simulink model "FM_V6_Zikun"  (R2022b)
settings: Solver=VariableStepAuto  StartTime=0.0  StopTime=1240
values from neighbouring files (symbols this model uses):
  A_fc = 550    [CNV.m]
  A_st = 1.1*A_fc*1E-4*n_cell*0.0012    (= 0.047553)    [CNV.m]
  A_T_rm = 0.005    [CNV.m]
  b11 = 0.005139    [CNV.m]
  b12 = 0.00326    [CNV.m]
  b2 = 350    [CNV.m]
  c1 = 10    [CNV.m]
  c3 = 2    [CNV.m]
  cc = 30    [CNV.m]
  Cd_rm = 0.0124    [CNV.m]
  Cp_air = 1005    [CNV.m]
  Cp_cl = 4180    [CNV.m]
  Cp_st = Cp_Al*1.5    (= 1350)    [CNV.m]
  F = 96485    [CNV.m]
  gamma = 1.4    [CNV.m]
  H_conv_st = 3    [CNV.m]
  i_max = 2.2    [CNV.m]
  k_ca_out = 0.2177*10^(-5)    (= 2.177e-06)    [CNV.m]
  K_sm_out = 0.3629*10^-5    (= 3.629e-06)    [CNV.m]
  kd_cp = 0.01    [CNV.m]
  kd_rm = 0    [CNV.m]
  ki_cp = 0.1    [CNV.m]
  ki_fan = -1E-5    (= -1e-05)    [CNV.m]
  ki_rm = -5E-8    (= -5e-08)    [CNV.m]
  kp_cp = 7.5    [CNV.m]
  kp_fan = -0.5    [CNV.m]
  kp_rm = -8E-7    (= -8e-07)    [CNV.m]
  M_a = 29*10^-3    (= 0.029)    [CNV.m]
  M_H2 = 2*10^-3    (= 0.002)    [CNV.m]
  m_H2_initial = P_atm*V_an/(R_H2*T_atm)    (= 0.00044494386048)    [CNV.m]
  m_H2O_initial = 0.005    [CNV.m]
  M_m_dry = 1.1    [CNV.m]
  M_N2 = 28*10^-3    (= 0.028)    [CNV.m]
  m_N2_initial = P_atm*(1-y_O2)*V_ca/(R_N2*T_atm)    (= 0.00586138039643)    [CNV.m]
  M_O2 = 32*10^-3    (= 0.032)    [CNV.m]
  m_O2_initial = P_atm*y_O2*V_ca/(R_O2*T_atm)    (= 0.00177998712422)    [CNV.m]
  m_st = n_cell*A_fc*t_m*rho_m_dry+(V_ca+V_an)*rho_Al*2.5    (= 87.4506875)    [CNV.m]
  M_v = 18*10^-3    (= 0.018)    [CNV.m]
  n_cell = 655    [CNV.m]
  P_a = P_atm*(1-L*h/T_atm)^(g*M_a/(R*L))    [CNV.m]
  P_atm = 101.25*10^3    (= 101250)    [CNV.m]
  P_ca_ref = 2.5*P_a    [CNV.m]
  phi_a = 0.1    [CNV.m]
  phi_des = 1    [CNV.m]
  R = 8.315    [CNV.m]
  R_a = 286.9    [CNV.m]
  R_H2 = 4124.3    [CNV.m]
  R_N2 = 296.8    [CNV.m]
  R_O2 = 259.8    [CNV.m]
  R_v = 461.5    [CNV.m]
  rho_a = P_a/(R_a*T_a)    [CNV.m]
  rho_H2 = 0.0899    [CNV.m]
  rho_m_dry = 0.002    [CNV.m]
  rho_N2 = 1.165    [CNV.m]
  T_a = T_atm-h*L    [CNV.m]
  T_atm = 298.15    [CNV.m]
  T_cl = 353.15    [CNV.m]
  t_m = 0.01    [CNV.m]
  T_rm = 303.15    [CNV.m]
  T_st_ref = 353.15    [CNV.m]
  V_an = n_cell*A_fc*10^(-4)*0.0005*0.3    (= 0.00540375)    [CNV.m]
  V_ca = n_cell*A_fc*10^(-4)*0.0006*0.3    (= 0.0064845)    [CNV.m]
  V_rm = 0.005    [CNV.m]
  V_sm = 0.02    [CNV.m]
  y_O2_ca_in = 0.21    [CNV.m]
libraries: fl_lib x64, nesl_utility x40, ee_lib x18, fl_ps_legacy_lib x6, SimscapeFluids_lib x5, slpidlib x4, simulink x3, batteryecm_lib x1, autolibshared x1
(part 5 of 6)

== system FM_V6_Zikun/Subsystem/FuelCellStack1/MembraneHydration ==
  I_st : Inport
  T_st : Inport  Port=2
  phi_ca : Inport  Port=3
  phi_an : Inport  Port=4
  3.67-3.70 : MATLAB Function  TreatAsAtomicUnit=on
  3.72-3.73 : MATLAB Function  TreatAsAtomicUnit=on
  3.74 : MATLAB Function  TreatAsAtomicUnit=on
  3.75-3.76 : MATLAB Function  TreatAsAtomicUnit=on
  3.77-3.78 : Gain  Gain=rho_m_dry/M_m_dry
  Add : Sum
  Constant : Constant  Value=n_cell
  Constant1 : Constant  Value=M_v
  Constant2 : Constant  Value=A_fc
  Constant3 : Constant  Value=t_m
  Constant4 : Constant  Value=F
  Demux : Demux  Outputs=2
  Gain : Gain  Gain=1/A_fc
  Mux : Mux  Inputs=2
  Scope : Scope
  lambda_m : Outport
  W_v_mem : Outport  Port=2
  wires:
  Mux/1 -> 3.77-3.78/1
  Demux/1 -> 3.67-3.70/4(c_v_ca)
  Demux/2 -> 3.67-3.70/5(c_v_an)
  3.72-3.73/2(lambda_ca) -> Mux/1
  3.72-3.73/3(lambda_an) -> Mux/2
  3.77-3.78/1 -> Demux/1
  I_st/1 -> Gain/1
  phi_ca/1 -> Add/1, 3.72-3.73/1(phi_ca)
  phi_an/1 -> Add/2, 3.72-3.73/2(phi_an)
  3.67-3.70/1(W_v_mem) -> W_v_mem/1
  3.72-3.73/1(lambda_m) -> 3.74/1(lambda_m), 3.75-3.76/1(lambda_m), lambda_m/1
  3.74/1(n_d) -> 3.67-3.70/1(n_d)
  3.75-3.76/1(D_w) -> 3.67-3.70/3(D_w)
  T_st/1 -> 3.75-3.76/2(T_st)
  Gain/1 -> 3.67-3.70/2(i)
  Constant/1 -> 3.67-3.70/6(n_cell)
  Constant1/1 -> 3.67-3.70/8(M_v)
  Constant2/1 -> 3.67-3.70/7(A_fc)
  Constant3/1 -> 3.67-3.70/9(t_m)
  Constant4/1 -> 3.67-3.70/10(F)
  Add/1 -> Scope/1

== system FM_V6_Zikun/Subsystem/FuelCellStack1/StackVoltage ==
  P_ca : Inport
  P_O2 : Inport  Port=2
  lambda_m : Inport  Port=3
  P_H2 : Inport  Port=4
  P_sat : Inport  Port=5
  T_st : Inport  Port=6
  I_st : Inport  Port=7
  ActivationLoss : Subsystem
  ConcentrationLoss : Subsystem
  Constant : Constant  Value=n_cell
  Demux : Demux
  Gain : Gain  Gain=1/A_fc
  MATLAB Function : MATLAB Function  TreatAsAtomicUnit=on
  Mux : Mux
  NernstVoltage : MATLAB Function  TreatAsAtomicUnit=on
  OhmicLoss : Subsystem
  Pa2Bar : Gain  Gain=0.00001
  Product : Product
  Scope1 : Scope  NumInputPorts=5
  Scope2 : Scope
  Scope3 : Scope  NumInputPorts=4
  To Workspace : ToWorkspace  VariableName=simout  SaveFormat=Timeseries  SampleTime=-1
  VoltageBehaviour : Subsystem  Commented=on
  StackVoltage : Outport
  tag scope: CellVoltage=global, I_den=global
  wires:
  ConcentrationLoss/1(V_conc) -> MATLAB Function/4(V_conc), Scope1/4
  MATLAB Function/1(V_cell) -> Scope1/5, [CellVoltage], Product/1, Scope2/1, To Workspace/1  "V_cell"
  OhmicLoss/1(V_ohm) -> MATLAB Function/3(V_ohm), Scope1/3
  Constant/1 -> Product/2
  Product/1 -> StackVoltage/1
  NernstVoltage/1(E_T_P) -> MATLAB Function/1(E_T_P), Scope1/1
  ActivationLoss/1(V_act) -> MATLAB Function/2(V_act), Scope1/2
  T_st/1 -> ConcentrationLoss/2(T_st), OhmicLoss/2(T_st), ActivationLoss/1(T_st), NernstVoltage/1(T_st)
  lambda_m/1 -> OhmicLoss/3(lambda_m)
  I_st/1 -> Gain/1
  Gain/1 -> [I_den], ConcentrationLoss/1(I_den), ActivationLoss/5(I_den), OhmicLoss/1(I_den)
  P_H2/1 -> Mux/1
  P_O2/1 -> Mux/2
  P_sat/1 -> Mux/4
  Mux/1 -> Pa2Bar/1
  Demux/1 -> NernstVoltage/2(P_H2)
  Demux/2 -> ActivationLoss/4(P_O2), ConcentrationLoss/3(P_O2), NernstVoltage/3(P_O2)
  Demux/3 -> ActivationLoss/2(P_ca)
  Demux/4 -> ConcentrationLoss/4(P_sat), ActivationLoss/3(P_sat)
  Pa2Bar/1 -> Demux/1
  P_ca/1 -> Mux/3

== system FM_V6_Zikun/Subsystem/FuelCellStack1/Thermo ==
  Constant : Constant  Value=n_cell
  MATLAB Function : MATLAB Function  TreatAsAtomicUnit=on
  Scope : Scope  NumInputPorts=2
  wires:
  [I_st] -> MATLAB Function/1(I_st)
  Constant/1 -> MATLAB Function/3(n_cell)
  [CellVoltage] -> MATLAB Function/2(V_cell)
  MATLAB Function/1(P_loss_reac) -> Scope/1
  [P_st] -> Scope/2

== system FM_V6_Zikun/Subsystem/Subsystem2/Subsystem ==
  T_cl_in : Inport
  I_st : Inport  Port=2
  Constant : Constant  Value=0.3
  Constant1 : Constant  Value=Cp_air
  Constant2 : Constant  Value=Cp_cl
  Constant3 : Constant  Value=T_a
  Constant4 : Constant  Value=T_st_ref
  Constant5 : Constant  Value=0
  Constant6 : Constant  Value=10
  Demux : Demux  Outputs=2
  MATLAB Function : MATLAB Function  TreatAsAtomicUnit=on
  MATLAB Function1 : MATLAB Function  TreatAsAtomicUnit=on
  MATLAB Function3 : MATLAB Function  TreatAsAtomicUnit=on
  Minus : Sum  Inputs=+-
  Mux : Mux  Inputs=2
  Mux1 : Mux  Inputs=2
  PID Controller1 : slpidlib/PID Controller  Controller=PID  Form=Parallel  TimeDomain=Continuous-time  UseExternalTs=off  SampleTime=-1  IntegratorMethod=Forward Euler  FilterMethod=Forward Euler  ControllerParametersSource=internal  P=kp_fan  I=ki_fan  UseKiTs=off  D=0  N=100  UseFilter=on  TunerSelectOption=Transfer Function Based (PID Tuner App)  InitialConditionSource=internal  InitialConditionForIntegrator=0  InitialConditionForFilter=0  DifferentiatorICPrevScaledInput=0  ExternalReset=none  TrackingMode=off  Kt=1  LimitOutput=off  SatLimitsSource=internal  UpperSaturationLimit=inf  LowerSaturationLimit=-inf  LinearizeAsGain=on  AntiWindupMode=none  Kb=1  LimitIntegrator=off  UpperIntegratorSaturationLimit=inf  LowerIntegratorSaturationLimit=-inf  POutMin=[]  POutMax=[]  IOutMin=[]  IOutMax=[]  DOutMin=[]  DOutMax=[]  NOutMin=[]  NOutMax=[]  SumOutMin=[]  SumOutMax=[]  SaturationOutMin=[]  SaturationOutMax=[]  PParamMin=[]  PParamMax=[]  IParamMin=[]  IParamMax=[]  DParamMin=[]  DParamMax=[]  NParamMin=[]  NParamMax=[]  KbParamMin=[]  KbParamMax=[]  KtParamMin=[]  KtParamMax=[]  KbOutMin=[]  KbOutMax=[]  KtOutMin=[]  KtOutMax=[]  IntegratorOutMin=[]  IntegratorOutMax=[]  FilterOutMin=[]  FilterOutMax=[]  SumI1OutMin=[]  SumI1OutMax=[]  SumI2OutMin=[]  SumI2OutMax=[]  SumI3OutMin=[]  SumI3OutMax=[]  SumI4OutMin=[]  SumI4OutMax=[]  SumDOutMin=[]  SumDOutMax=[]  DifferentiatorOutMin=[]  DifferentiatorOutMax=[]  FilterDiffOutCoefMin=[]  FilterDiffOutCoefMax=[]  ReciprocalOutMin=[]  ReciprocalOutMax=[]  SumDenOutMin=[]  SumDenOutMax=[]  SumNumOutMin=[]  SumNumOutMax=[]  DivideOutMin=[]  DivideOutMax=[]  UdiffTsProdOutMin=[]  UdiffTsProdOutMax=[]  NTsProdOutMin=[]  NTsProdOutMax=[]  UintegralTsProdOutMin=[]  UintegralTsProdOutMax=[]  UngainTsProdOutMin=[]  UngainTsProdOutMax=[]  ClampingZeroOutDataTypeStr=Inherit: Inherit via back propagation  ClampingZeroOutMin=[]  ClampingZeroOutMax=[]  FilterDenConstantOutDataTypeStr=Inherit: Inherit via back propagation  FilterDenConstantOutMin=[]  FilterDenConstantOutMax=[]  PCopyOutDataTypeStr=Inherit: Inherit via back propagation  PCopyOutMin=[]  PCopyOutMax=[]  NCopyOutDataTypeStr=Inherit: Inherit via back propagation  NCopyOutMin=[]  NCopyOutMax=[]  IntegratorContinuousStateAttributes=''  IntegratorStateMustResolveToSignalObject=off  IntegratorRTWStateStorageClass=Auto  FilterContinuousStateAttributes=''  FilterStateMustResolveToSignalObject=off  FilterRTWStateStorageClass=Auto  ParallelPVariant=InternalParameters  IdealPVariant=Disabled  IVariant=InternalParameters  DVariant=InternalParameters  IntegratorVariant=Continuous  SatVariant=Disabled  AWVariant=Passthrough  PCopyVariant=Disabled  TRVariant=Disabled  FdbkBlocksVariant=Forward  IdealPFdbkVariant=Disabled  SatFdbkVariant=Disabled  DerivativeFilterVariant=ContFilter  NVariant=InternalParameters  NCopyVariant=Disabled  FilterICVariant=InternalICsFilter  IntegratorICVariant=InternalICs  ExternalResetVariant=Disabled  TRSumVariant=Passthrough  SumFdbkVariant=Disabled  SumVariant=Sum_PID  TsampFilterVariant=InternalTs  TsampNgainVariant=Passthrough  TsampIntegralVariant=Passthrough  ExternalSaturationOutDataTypeStr=Inherit: Same as second input
  PID Controller2 : slpidlib/PID Controller  Controller=PID  Form=Parallel  TimeDomain=Continuous-time  UseExternalTs=off  SampleTime=-1  IntegratorMethod=Forward Euler  FilterMethod=Forward Euler  ControllerParametersSource=internal  P=-0.5  I=-1E-3  UseKiTs=off  D=0  N=100  UseFilter=on  TunerSelectOption=Transfer Function Based (PID Tuner App)  InitialConditionSource=internal  InitialConditionForIntegrator=0  InitialConditionForFilter=0  DifferentiatorICPrevScaledInput=0  ExternalReset=none  TrackingMode=off  Kt=1  LimitOutput=off  SatLimitsSource=internal  UpperSaturationLimit=inf  LowerSaturationLimit=-inf  LinearizeAsGain=on  AntiWindupMode=none  Kb=1  LimitIntegrator=off  UpperIntegratorSaturationLimit=inf  LowerIntegratorSaturationLimit=-inf  POutMin=[]  POutMax=[]  IOutMin=[]  IOutMax=[]  DOutMin=[]  DOutMax=[]  NOutMin=[]  NOutMax=[]  SumOutMin=[]  SumOutMax=[]  SaturationOutMin=[]  SaturationOutMax=[]  PParamMin=[]  PParamMax=[]  IParamMin=[]  IParamMax=[]  DParamMin=[]  DParamMax=[]  NParamMin=[]  NParamMax=[]  KbParamMin=[]  KbParamMax=[]  KtParamMin=[]  KtParamMax=[]  KbOutMin=[]  KbOutMax=[]  KtOutMin=[]  KtOutMax=[]  IntegratorOutMin=[]  IntegratorOutMax=[]  FilterOutMin=[]  FilterOutMax=[]  SumI1OutMin=[]  SumI1OutMax=[]  SumI2OutMin=[]  SumI2OutMax=[]  SumI3OutMin=[]  SumI3OutMax=[]  SumI4OutMin=[]  SumI4OutMax=[]  SumDOutMin=[]  SumDOutMax=[]  DifferentiatorOutMin=[]  DifferentiatorOutMax=[]  FilterDiffOutCoefMin=[]  FilterDiffOutCoefMax=[]  ReciprocalOutMin=[]  ReciprocalOutMax=[]  SumDenOutMin=[]  SumDenOutMax=[]  SumNumOutMin=[]  SumNumOutMax=[]  DivideOutMin=[]  DivideOutMax=[]  UdiffTsProdOutMin=[]  UdiffTsProdOutMax=[]  NTsProdOutMin=[]  NTsProdOutMax=[]  UintegralTsProdOutMin=[]  UintegralTsProdOutMax=[]  UngainTsProdOutMin=[]  UngainTsProdOutMax=[]  ClampingZeroOutDataTypeStr=Inherit: Inherit via back propagation  ClampingZeroOutMin=[]  ClampingZeroOutMax=[]  FilterDenConstantOutDataTypeStr=Inherit: Inherit via back propagation  FilterDenConstantOutMin=[]  FilterDenConstantOutMax=[]  PCopyOutDataTypeStr=Inherit: Inherit via back propagation  PCopyOutMin=[]  PCopyOutMax=[]  NCopyOutDataTypeStr=Inherit: Inherit via back propagation  NCopyOutMin=[]  NCopyOutMax=[]  IntegratorContinuousStateAttributes=''  IntegratorStateMustResolveToSignalObject=off  IntegratorRTWStateStorageClass=Auto  FilterContinuousStateAttributes=''  FilterStateMustResolveToSignalObject=off  FilterRTWStateStorageClass=Auto  ParallelPVariant=InternalParameters  IdealPVariant=Disabled  IVariant=InternalParameters  DVariant=InternalParameters  IntegratorVariant=Continuous  SatVariant=Disabled  AWVariant=Passthrough  PCopyVariant=Disabled  TRVariant=Disabled  FdbkBlocksVariant=Forward  IdealPFdbkVariant=Disabled  SatFdbkVariant=Disabled  DerivativeFilterVariant=ContFilter  NVariant=InternalParameters  NCopyVariant=Disabled  FilterICVariant=InternalICsFilter  IntegratorICVariant=InternalICs  ExternalResetVariant=Disabled  TRSumVariant=Passthrough  SumFdbkVariant=Disabled  SumVariant=Sum_PID  TsampFilterVariant=InternalTs  TsampNgainVariant=Passthrough  TsampIntegralVariant=Passthrough  ExternalSaturationOutDataTypeStr=Inherit: Same as second input
  Plus : Sum  Inputs=+-
  Saturation : Saturate  UpperLimit=5  LowerLimit=0
  Scope : Scope  NumInputPorts=2
  Switch : Switch  Criteria=u2 > Threshold  Threshold=20  SaturateOnIntegerOverflow=off  InputSameDT=off
  To Workspace1 : ToWorkspace  VariableName=W_cl_rad  SaveFormat=Timeseries  SampleTime=-1
  To Workspace7 : ToWorkspace  VariableName=W_air_rad  SaveFormat=Timeseries  SampleTime=-1
  P_pump_loss : Outport
  P_fan_loss : Outport  Port=2
  P_cl : Outport  Port=3
  wires:
  T_cl_in/1 -> MATLAB Function/3(T_cl_in), Plus/2, MATLAB Function3/2(T_st)
  Constant4/1 -> Minus/1, MATLAB Function3/1(T_st_ref)
  MATLAB Function1/2(P_pump_loss) -> P_pump_loss/1
  MATLAB Function1/1(P_fan_loss) -> P_fan_loss/1
  MATLAB Function/1(P_cl) -> P_cl/1
  Constant/1 -> MATLAB Function/4(nu_rad)
  Constant1/1 -> MATLAB Function/5(Cp_a)
  Constant2/1 -> MATLAB Function/6(Cp_cl)
  Constant3/1 -> MATLAB Function/7(T_a_in)
  MATLAB Function3/2(e_fan) -> PID Controller1/1
  PID Controller1/1 -> Mux/2
  MATLAB Function3/1(W_cl) -> Mux/1
  I_st/1 -> Switch/2
  Mux/1 -> Switch/1
  Demux/1 -> Saturation/1
  Demux/2 -> To Workspace7/1, MATLAB Function1/1(W_a), Scope/2, MATLAB Function/2(W_a)
  Switch/1 -> Demux/1
  Mux1/1 -> Switch/3
  Constant5/1 -> Mux1/2
  PID Controller2/1 -> Mux1/1
  Plus/1 -> PID Controller2/1
  Saturation/1 -> To Workspace1/1, MATLAB Function1/2(W_cl), Scope/1, MATLAB Function/1(W_cl)
  Minus/1 -> Plus/1
  Constant6/1 -> Minus/2

== system FM_V6_Zikun/Subsystem/Subsystem2/ThermoCalc ==
  I_st : Inport
  P_st : Inport  Port=2
  P_cl : Inport  Port=3
  Add : Sum  Inputs=+---
  Constant : Constant  Value=F
  Constant1 : Constant  Value=n_cell
  Constant2 : Constant  Value=T_a
  Constant6 : Constant  Value=H_conv_st
  Constant7 : Constant  Value=A_st
  Gain : Gain  Gain=1/(m_st*Cp_st)
  Integrator : Integrator  InitialCondition=T_a
  P_conv : MATLAB Function  TreatAsAtomicUnit=on
  P_tot : MATLAB Function  TreatAsAtomicUnit=on
  Saturation1 : Saturate  Commented=through  UpperLimit=400  LowerLimit=T_a
  Scope : Scope  NumInputPorts=4
  T_st : Outport
  P_tot_st : Outport  Port=2
  wires:
  P_cl/1 -> Scope/3, Add/3
  Constant6/1 -> P_conv/1(k_conv)
  Constant2/1 -> P_conv/3(T_a)
  P_st/1 -> Scope/2, Add/2
  Constant7/1 -> P_conv/2(A_st)
  Gain/1 -> Integrator/1
  Constant1/1 -> P_tot/3(n_cell)
  Integrator/1 -> P_conv/4(T_st), Saturation1/1
  P_conv/1(P_conv) -> Scope/4, Add/4
  Add/1 -> Gain/1
  P_tot/1(P_tot) -> Scope/1, Add/1, P_tot_st/1
  Constant/1 -> P_tot/2(F)
  I_st/1 -> P_tot/1(I_st)
  Saturation1/1 -> T_st/1

== system FM_V6_Zikun/Subsystem/Supply Manifold/Manifold Filling ==
  W_cp : Inport
  T_cp_out : Inport  Port=2
  W_sm_out : Inport  Port=3
  Constant : Constant  Value=T_atm
  Constant1 : Constant  Value=gamma
  Constant2 : Constant  Value=R_a
  Constant3 : Constant  Value=V_sm
  Integrator : Integrator  InitialCondition=P_atm
  Integrator1 : Integrator
  MATLAB Function : MATLAB Function  TreatAsAtomicUnit=on
  MATLAB Function1 : MATLAB Function  TreatAsAtomicUnit=on
  MATLAB Function2 : MATLAB Function  TreatAsAtomicUnit=on
  Switch : Switch  Criteria=u2 > Threshold  SaturateOnIntegerOverflow=off  InputSameDT=off
  p_sm : Outport
  T_sm : Outport  Port=2
  wires:
  W_cp/1 -> MATLAB Function1/1(W_cp), MATLAB Function/1(W_cp)
  T_cp_out/1 -> MATLAB Function1/2(T_cp_out)
  MATLAB Function1/1(d_p_sm_dt) -> Integrator/1
  MATLAB Function2/1(T_sm) -> Switch/1, Switch/2, T_sm/1
  Integrator/1 -> p_sm/1, MATLAB Function2/2(p_sm)
  MATLAB Function/1(d_m_sm_dt) -> Integrator1/1
  W_sm_out/1 -> MATLAB Function/2(W_sm_out), MATLAB Function1/3(W_sm_out)
  Integrator1/1 -> MATLAB Function2/1(m_sm)
  Constant/1 -> Switch/3
  Switch/1 -> MATLAB Function1/4(T_sm)
  Constant1/1 -> MATLAB Function1/5(gamma)
  Constant2/1 -> MATLAB Function1/6(R_a), MATLAB Function2/4(R_a)
  Constant3/1 -> MATLAB Function1/7(V_sm), MATLAB Function2/3(V_sm)

== system FM_V6_Zikun/Subsystem/Supply Manifold/Nozzle ==
  P_ca : Inport
  P_sm : Inport  Port=2
  Constant : Constant  Value=K_sm_out
  MATLAB Function : MATLAB Function  TreatAsAtomicUnit=on
  W_sm_out : Outport
  wires:
  P_sm/1 -> MATLAB Function/1(P_sm)
  P_ca/1 -> MATLAB Function/2(P_ca)
  MATLAB Function/1(W_sm_out) -> W_sm_out/1
  Constant/1 -> MATLAB Function/3(k_sm_out)

== system FM_V6_Zikun/D/Subsystem/Electric Pump System/Temperature measurement1 ==
  Tamb : Inport
  Convective Heat Transfer : fl_lib/Thermal/Thermal Elements/Convective Heat Transfer  thermal_type=foundation.enum.constant_variable.constant  area=0.1 m^2  heat_tr_coeff=5 W/(m^2 * K)  min_heat_tr_coeff=1e-3 W/(K*m^2)  T_specify=off  T_priority=None  T=0 K  T_nominal_specify=off  T_nominal_unit=K  T_nominal_value=1  Q_specify=off  Q_priority=None  Q=0 J/s  Q_nominal_specify=off  Q_nominal_unit=J/s  Q_nominal_value=1
  PS-Simulink Converter1 : nesl_utility/PS-Simulink Converter  PhysicalDomain=network_engine_domain  SubClassName=ps_output  LeftPortType=input  RightPortType=output  PseudoPeriodic=off  Frequencies=[]  VectorFormat=1-D array  Unit=degC  AffineConversion=on
  Simulink-PS Converter1 : nesl_utility/Simulink-PS Converter  PhysicalDomain=network_engine_domain  SubClassName=ps_input  LeftPortType=input  RightPortType=output  PseudoPeriodic=off  Frequencies=[]  NoiseDistribution=none  NoiseParameters=[]  Unit=degC  AffineConversion=on  FilteringAndDerivatives=zero  SimscapeFilterOrder=1  InputFilterTimeConstant=0.001  UdotUserProvided=1
  Temperature Sensor : fl_lib/Thermal/Thermal Sensors/Temperature Sensor
  Temperature Source : fl_lib/Thermal/Thermal Sources/Controlled Temperature Source
  Thermal Reference : fl_lib/Thermal/Thermal Elements/Thermal Reference
  H : PMIOPort  Side=Right
  T : Outport  VectorParamsAs1DForOutWhenUnconnected=off
  wires:
  Tamb/1 -> Simulink-PS Converter1/1
  PS-Simulink Converter1/1 -> T/1  "Temperature [degC]"
  connections:
  Convective Heat Transfer/RConn1 -- Temperature Source/LConn1
  Temperature Sensor/RConn2 -- PS-Simulink Converter1/LConn1
  Temperature Sensor/LConn1 -- H/RConn1 -- Convective Heat Transfer/LConn1
  Simulink-PS Converter1/RConn1 -- Temperature Source/RConn1
  Thermal Reference/LConn1 -- Temperature Sensor/RConn1 -- Temperature Source/RConn2

== system FM_V6_Zikun/D/Subsystem/Electric Pump System/Temperature measurement2 ==
  Tamb : Inport
  Convective Heat Transfer : fl_lib/Thermal/Thermal Elements/Convective Heat Transfer  thermal_type=foundation.enum.constant_variable.constant  area=0.1 m^2  heat_tr_coeff=5 W/(m^2 * K)  min_heat_tr_coeff=1e-3 W/(K*m^2)  T_specify=off  T_priority=None  T=0 K  T_nominal_specify=off  T_nominal_unit=K  T_nominal_value=1  Q_specify=off  Q_priority=None  Q=0 J/s  Q_nominal_specify=off  Q_nominal_unit=J/s  Q_nominal_value=1
  PS-Simulink Converter1 : nesl_utility/PS-Simulink Converter  PhysicalDomain=network_engine_domain  SubClassName=ps_output  LeftPortType=input  RightPortType=output  PseudoPeriodic=off  Frequencies=[]  VectorFormat=1-D array  Unit=degC  AffineConversion=on
  Simulink-PS Converter1 : nesl_utility/Simulink-PS Converter  PhysicalDomain=network_engine_domain  SubClassName=ps_input  LeftPortType=input  RightPortType=output  PseudoPeriodic=off  Frequencies=[]  NoiseDistribution=none  NoiseParameters=[]  Unit=degC  AffineConversion=on  FilteringAndDerivatives=zero  SimscapeFilterOrder=1  InputFilterTimeConstant=0.001  UdotUserProvided=1
  Temperature Sensor : fl_lib/Thermal/Thermal Sensors/Temperature Sensor
  Temperature Source : fl_lib/Thermal/Thermal Sources/Controlled Temperature Source
  Thermal Reference : fl_lib/Thermal/Thermal Elements/Thermal Reference
  H : PMIOPort  Side=Right
  T : Outport  VectorParamsAs1DForOutWhenUnconnected=off
  wires:
  Tamb/1 -> Simulink-PS Converter1/1
  PS-Simulink Converter1/1 -> T/1  "Temperature [degC]"
  connections:
  Convective Heat Transfer/RConn1 -- Temperature Source/LConn1
  Temperature Sensor/RConn2 -- PS-Simulink Converter1/LConn1
  Temperature Sensor/LConn1 -- H/RConn1 -- Convective Heat Transfer/LConn1
  Simulink-PS Converter1/RConn1 -- Temperature Source/RConn1
  Thermal Reference/LConn1 -- Temperature Sensor/RConn1 -- Temperature Source/RConn2

== system FM_V6_Zikun/Subsystem/Compressor/Subsystem/Subsystem1 ==
  P_ca : Inport
  Add : Sum  Inputs=+-
  Add1 : Sum  Inputs=+++
  Constant : Constant  Value=P_ca_ref
  Derivative : Derivative
  Gain : Gain  Gain=0.000001
  Gain1 : Gain  Gain=0
  Gain2 : Gain  Gain=0
  Integrator : Integrator
  Scope : Scope
  diff : Outport
  wires:
  P_ca/1 -> Add/2
  Constant/1 -> Add/1
  Add/1 -> Scope/1, Derivative/1, Integrator/1, Gain/1
  Gain/1 -> Add1/1
  Gain1/1 -> Add1/2
  Gain2/1 -> Add1/3
  Integrator/1 -> Gain1/1
  Derivative/1 -> Gain2/1
  Add1/1 -> diff/1

== system FM_V6_Zikun/Subsystem/FuelCellStack1/Anode Flow Model/Diffusion ==
  P_an : Inport
  W_H2_an_in : Inport  Port=2
  T_st : Inport  Port=3
  Constant : Constant  Value=A_fc
  Constant1 : Constant  Value=t_m
  Constant2 : Constant  Value=n_cell
  H2 Crossflow : MATLAB Function  TreatAsAtomicUnit=on
  W_H2_an_cf : Outport
  W_H2_an_in2 : Outport  Port=2
  wires:
  P_an/1 -> H2 Crossflow/4(P_an)
  T_st/1 -> H2 Crossflow/6(T_st)
  Constant2/1 -> H2 Crossflow/1(n_cell)
  Constant/1 -> H2 Crossflow/2(A_fc)
  Constant1/1 -> H2 Crossflow/3(t_m)
  H2 Crossflow/2(W_H2_an_in2) -> W_H2_an_in2/1
  H2 Crossflow/1(W_H2_an_cf) -> W_H2_an_cf/1
  W_H2_an_in/1 -> H2 Crossflow/5(W_H2_an_in)

== system FM_V6_Zikun/Subsystem/FuelCellStack1/Anode Flow Model/InletFlow ==
  P_v_an_in : Inport
  W_an_in : Inport  Port=2
  P_an_in : Inport  Port=3
  I_st : Inport  Port=4
  Constant : Constant  Value=n_cell
  Constant1 : Constant  Value=M_v
  Constant2 : Constant  Value=F
  Constant3 : Constant  Value=M_H2
  Minus : Sum  Inputs=+-
  Scope{,1..3} (4 alike) : Scope
  anode humidity ratio (3.62) : MATLAB Function  TreatAsAtomicUnit=on
  mass flow rates of hydrogen (3.63) : MATLAB Function  TreatAsAtomicUnit=on
  rate of hydrogen consumed in the reaction (3.65) : MATLAB Function  TreatAsAtomicUnit=on
  W_H2_an_in : Outport
  W_v_an_in : Outport  Port=2
  W_H2_reacted : Outport  Port=3
  tag scope: w_an_in=global
  wires:
  I_st/1 -> rate of hydrogen consumed in the reaction (3.65)/1(I_st)
  P_v_an_in/1 -> anode humidity ratio (3.62)/1(P_v_an_in)
  W_an_in/1 -> Scope3/1, mass flow rates of hydrogen (3.63)/2(W_an_in), Minus/1
  P_an_in/1 -> anode humidity ratio (3.62)/2(P_an_in)
  rate of hydrogen consumed in the reaction (3.65)/1(W_H2_reacted) -> Scope1/1, W_H2_reacted/1
  anode humidity ratio (3.62)/1(w_an_in) -> [w_an_in], mass flow rates of hydrogen (3.63)/1(w_an_in)
  Minus/1 -> Scope2/1, W_v_an_in/1
  Constant/1 -> rate of hydrogen consumed in the reaction (3.65)/2(n_cell)
  Constant3/1 -> anode humidity ratio (3.62)/4(M_H2), rate of hydrogen consumed in the reaction (3.65)/3(M_H2)
  Constant1/1 -> anode humidity ratio (3.62)/3(M_v)
  Constant2/1 -> rate of hydrogen consumed in the reaction (3.65)/4(F)
  mass flow rates of hydrogen (3.63)/1(W_H2_an_in) -> Scope/1, W_H2_an_in/1, Minus/2

== system FM_V6_Zikun/Subsystem/FuelCellStack1/Anode Flow Model/MassBalance ==
  W_H2_an_in : Inport
  W_v_an_in : Inport  Port=2
  W_H2_reacted : Inport  Port=3
  W_v_mem : Inport  Port=4
  W_l_an_out : Inport  Port=5
  T_st : Inport  Port=6
  p_sat_tst : Inport  Port=7
  W_v_an_out : Inport  Port=8
  W_H2_an_out : Inport  Port=9
  3.51 : MATLAB Function  TreatAsAtomicUnit=on
  3.52 : MATLAB Function  TreatAsAtomicUnit=on
  3.53 & 3.54 : MATLAB Function  TreatAsAtomicUnit=on
  Constant : Constant  Value=V_an
  Constant1 : Constant  Value=R_v
  Integrator : Integrator  InitialCondition=0.001
  Integrator1 : Integrator  InitialCondition=m_H2_initial
  Scope{,1..3} (4 alike) : Scope
  maximum vapor mass (3.55) : MATLAB Function  TreatAsAtomicUnit=on
  m_H2_an : Outport
  m_v_an : Outport  Port=2
  m_l_an : Outport  Port=3
  wires:
  p_sat_tst/1 -> maximum vapor mass (3.55)/1(p_sat_tst)
  T_st/1 -> maximum vapor mass (3.55)/2(T_st)
  W_v_an_in/1 -> 3.52/1(W_v_an_in)
  3.53 & 3.54/1(m_v_an) -> m_v_an/1
  3.52/1(dm_w_an) -> Integrator/1
  Integrator/1 -> 3.53 & 3.54/2(m_w_an)
  3.53 & 3.54/2(m_l_an) -> m_l_an/1
  W_v_an_out/1 -> 3.52/2(W_v_an_out)
  W_H2_an_in/1 -> Scope1/1, 3.51/1(W_H2_an_in)
  W_H2_an_out/1 -> Scope2/1, 3.51/2(W_H2_an_out)
  W_H2_reacted/1 -> Scope3/1, 3.51/3(W_H2_reac)
  W_v_mem/1 -> 3.52/3(W_v_mem)
  W_l_an_out/1 -> 3.52/4(W_l_an_out)
  Constant/1 -> maximum vapor mass (3.55)/3(V_an)
  Constant1/1 -> maximum vapor mass (3.55)/4(R_v)
  Integrator1/1 -> m_H2_an/1
  3.51/1(dm_H2_an) -> Scope/1, Integrator1/1
  maximum vapor mass (3.55)/1(m_v_max_an) -> 3.53 & 3.54/1(m_v_max_an)

== system FM_V6_Zikun/Subsystem/FuelCellStack1/Anode Flow Model/OutletFlow ==
  W_an_out : Inport
  P_H2_an : Inport  Port=2
  P_v_an : Inport  Port=3
  3,66a : MATLAB Function  TreatAsAtomicUnit=on
  Constant : Constant  Value=M_v
  Constant1 : Constant  Value=M_H2
  outlet hydrogen mass flow rate (3.66b) : MATLAB Function  TreatAsAtomicUnit=on
  outlet vapor mass flow rate (3.66c) : MATLAB Function  TreatAsAtomicUnit=on
  W_v_an_out : Outport
  W_H2_an_out : Outport  Port=2
  wires:
  W_an_out/1 -> outlet vapor mass flow rate (3.66c)/1(W_an_out), outlet hydrogen mass flow rate (3.66b)/2(W_an_out)
  P_H2_an/1 -> 3,66a/2(P_H2_an)
  P_v_an/1 -> 3,66a/1(P_v_an)
  3,66a/1(w_an_out) -> outlet hydrogen mass flow rate (3.66b)/1(w_an_out)
  outlet hydrogen mass flow rate (3.66b)/1(W_H2_an_out) -> outlet vapor mass flow rate (3.66c)/2(W_H2_an_out), W_H2_an_out/1
  outlet vapor mass flow rate (3.66c)/1(W_v_an_out) -> W_v_an_out/1
  Constant/1 -> 3,66a/3(M_v)
  Constant1/1 -> 3,66a/4(M_H2)

== system FM_V6_Zikun/Subsystem/FuelCellStack1/Anode Flow Model/PsatCalc ==
  T_st : Inport
  T_an_in : Inport  Port=2
  PsatCalc (2.31) : MATLAB Function  TreatAsAtomicUnit=on
  PsatCalc1 (2.31) : MATLAB Function  TreatAsAtomicUnit=on
  P_sat_tst : Outport
  P_sat_t_an_in : Outport  Port=2
  wires:
  PsatCalc (2.31)/1(P_sat_tst) -> P_sat_tst/1
  T_st/1 -> PsatCalc (2.31)/1(T_st)
  T_an_in/1 -> PsatCalc1 (2.31)/1(T_an_in)
  PsatCalc1 (2.31)/1(P_sat_t_an_in) -> P_sat_t_an_in/1

== system FM_V6_Zikun/Subsystem/FuelCellStack1/Anode Flow Model/Subsystem1 ==
  phi_an_in : Inport
  p_sat_t_an_in : Inport  Port=2
  p_an_in : Inport  Port=3
  hydrogen partial pressure of the inlet flow (3.61) : Sum  Inputs=+-
  vapor pressure (3.60) : MATLAB Function  TreatAsAtomicUnit=on
  p_H2_an_in : Outport
  p_v_an_in : Outport  Port=2
  wires:
  p_sat_t_an_in/1 -> vapor pressure (3.60)/2(p_sat_t_an_in)
  phi_an_in/1 -> vapor pressure (3.60)/1(phi_an_in)
  p_an_in/1 -> hydrogen partial pressure of the inlet flow (3.61)/1
  vapor pressure (3.60)/1(p_v_an_in) -> p_v_an_in/1, hydrogen partial pressure of the inlet flow (3.61)/2
  hydrogen partial pressure of the inlet flow (3.61)/1 -> p_H2_an_in/1

== system FM_V6_Zikun/Subsystem/FuelCellStack1/Anode Flow Model/ThermodynamicCalc ==
  m_H2_an : Inport
  m_v_an : Inport  Port=2
  P_sat(T_st) : Inport  Port=3
  T_st : Inport  Port=4
  m_O2_an : Inport  Port=5
  m_N2_an : Inport  Port=6
  3.56 : MATLAB Function  TreatAsAtomicUnit=on
  3.56/3.57 N2 : MATLAB Function  TreatAsAtomicUnit=on
  3.56/3.57 O2 : MATLAB Function  TreatAsAtomicUnit=on
  3.57 : MATLAB Function  TreatAsAtomicUnit=on
  3.58 : Sum  Inputs=++++
  3.59 : Product  Inputs=*/
  Constant : Constant  Value=R_H2
  Constant1 : Constant  Value=V_an
  Constant2 : Constant  Value=R_v
  Constant3 : Constant  Value=R_O2
  Constant4 : Constant  Value=R_N2
  P_H2_an : Outport
  P_an : Outport  Port=2
  Phi_an : Outport  Port=3
  P_v_an : Outport  Port=4
  wires:
  3.57/1(P_v_an) -> P_v_an/1, 3.59/1, 3.58/2
  3.59/1 -> Phi_an/1
  3.58/1 -> P_an/1
  P_sat(T_st)/1 -> 3.59/2
  3.56/1(P_H2_an) -> P_H2_an/1, 3.58/1
  T_st/1 -> 3.56/3.57 N2/2(T_st), 3.56/3.57 O2/2(T_st), 3.57/2(T_st), 3.56/2(T_st)
  m_H2_an/1 -> 3.56/1(m_H2_an)
  m_v_an/1 -> 3.57/1(m_v_an)
  Constant/1 -> 3.56/4(R_H2)
  Constant1/1 -> 3.56/3.57 N2/3(V_an), 3.56/3.57 O2/3(V_an), 3.56/3(V_an), 3.57/3(V_an)
  Constant2/1 -> 3.57/4(R_v)
  m_O2_an/1 -> 3.56/3.57 O2/1(m_O2_an)
  m_N2_an/1 -> 3.56/3.57 N2/1(m_N2_an)
  Constant3/1 -> 3.56/3.57 O2/4(R_O2)
  Constant4/1 -> 3.56/3.57 N2/4(R_N2)
  3.56/3.57 O2/1(P_O2_an) -> 3.58/3
  3.56/3.57 N2/1(P_N2_an) -> 3.58/4

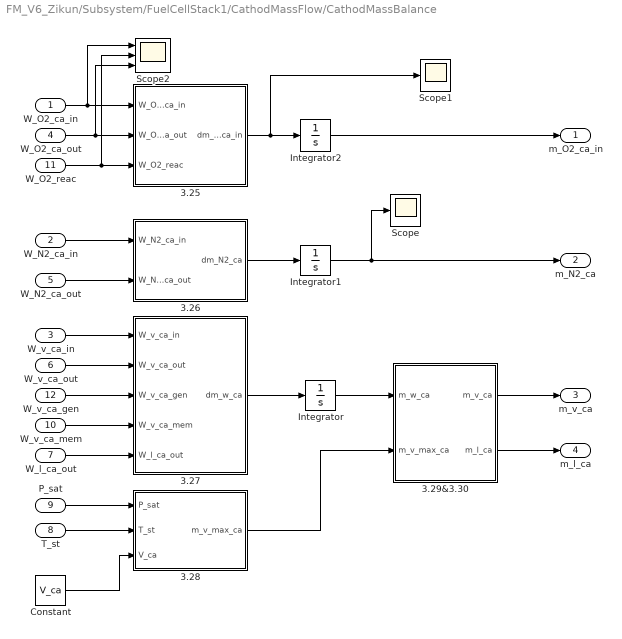
== system FM_V6_Zikun/Subsystem/FuelCellStack1/CathodMassFlow/CathodMassBalance ==
  W_O2_ca_in : Inport
  W_N2_ca_in : Inport  Port=2
  W_v_ca_in : Inport  Port=3
  W_O2_ca_out : Inport  Port=4
  W_N2_ca_out : Inport  Port=5
  W_v_ca_out : Inport  Port=6
  W_l_ca_out : Inport  Port=7
  T_st : Inport  Port=8
  P_sat : Inport  Port=9
  W_v_ca_mem : Inport  Port=10
  W_O2_reac : Inport  Port=11
  W_v_ca_gen : Inport  Port=12
  3.25 : MATLAB Function  TreatAsAtomicUnit=on
  3.26 : MATLAB Function  TreatAsAtomicUnit=on
  3.27 : MATLAB Function  TreatAsAtomicUnit=on
  3.28 : MATLAB Function  TreatAsAtomicUnit=on
  3.29&3.30 : MATLAB Function  TreatAsAtomicUnit=on
  Constant : Constant  Value=V_ca
  Integrator : Integrator  InitialCondition=m_H2O_initial
  Integrator1 : Integrator  InitialCondition=m_N2_initial
  Integrator2 : Integrator  InitialCondition=m_O2_initial
  Scope : Scope
  Scope1 : Scope
  Scope2 : Scope  NumInputPorts=3
  m_O2_ca_in : Outport
  m_N2_ca : Outport  Port=2
  m_v_ca : Outport  Port=3
  m_l_ca : Outport  Port=4
  wires:
  3.25/1(dm_O2_ca_in) -> Scope1/1, Integrator2/1
  3.26/1(dm_N2_ca) -> Integrator1/1
  3.27/1(dm_w_ca) -> Integrator/1
  Integrator2/1 -> m_O2_ca_in/1
  Integrator1/1 -> Scope/1, m_N2_ca/1
  Integrator/1 -> 3.29&3.30/1(m_w_ca)
  3.28/1(m_v_max_ca) -> 3.29&3.30/2(m_v_max_ca)
  3.29&3.30/1(m_v_ca) -> m_v_ca/1
  3.29&3.30/2(m_l_ca) -> m_l_ca/1
  W_O2_ca_in/1 -> Scope2/1, 3.25/1(W_O2_ca_in)
  W_N2_ca_in/1 -> 3.26/1(W_N2_ca_in)
  W_v_ca_in/1 -> 3.27/1(W_v_ca_in)
  W_O2_ca_out/1 -> Scope2/3, 3.25/2(W_O2_ca_out)
  W_N2_ca_out/1 -> 3.26/2(W_N2_ca_out)
  W_v_ca_out/1 -> 3.27/2(W_v_ca_out)
  W_l_ca_out/1 -> 3.27/5(W_l_ca_out)
  W_O2_reac/1 -> Scope2/2, 3.25/3(W_O2_reac)
  W_v_ca_gen/1 -> 3.27/3(W_v_ca_gen)
  W_v_ca_mem/1 -> 3.27/4(W_v_ca_mem)
  P_sat/1 -> 3.28/1(P_sat)
  T_st/1 -> 3.28/2(T_st)
  Constant/1 -> 3.28/3(V_ca)

== system FM_V6_Zikun/Subsystem/FuelCellStack1/CathodMassFlow/Diffusion ==
  lambda_m : Inport
  P_ca : Inport  Port=2
  W_O2_ca_in : Inport  Port=3
  W_N2_ca_in : Inport  Port=4
  T_st : Inport  Port=5
  Constant : Constant  Value=t_m
  Constant1 : Constant  Value=R
  Constant2 : Constant  Value=A_fc
  Constant3 : Constant  Value=n_cell
  O2 and N2 Crossflow : MATLAB Function  TreatAsAtomicUnit=on
  W_O2_ca_cf : Outport
  W_N2_ca_cf : Outport  Port=2
  W_O2_ca_in2 : Outport  Port=3
  W_N2_ca_in2 : Outport  Port=4
  wires:
  Constant/1 -> O2 and N2 Crossflow/3(t_m)
  Constant3/1 -> O2 and N2 Crossflow/1(n_cell)
  Constant2/1 -> O2 and N2 Crossflow/2(A_fc)
  P_ca/1 -> O2 and N2 Crossflow/4(P_ca)
  W_O2_ca_in/1 -> O2 and N2 Crossflow/5(W_O2_ca_in)
  W_N2_ca_in/1 -> O2 and N2 Crossflow/6(W_N2_ca_in)
  T_st/1 -> O2 and N2 Crossflow/7(T_st)
  O2 and N2 Crossflow/1(W_O2_ca_cf) -> W_O2_ca_cf/1
  O2 and N2 Crossflow/2(W_O2_ca_in2) -> W_O2_ca_in2/1
  O2 and N2 Crossflow/3(W_N2_ca_cf) -> W_N2_ca_cf/1
  O2 and N2 Crossflow/4(W_N2_ca_in2) -> W_N2_ca_in2/1
  Constant1/1 -> O2 and N2 Crossflow/9(R)
  lambda_m/1 -> O2 and N2 Crossflow/8(lambda_m)

== system FM_V6_Zikun/Subsystem/FuelCellStack1/CathodMassFlow/ElectroChemistry ==
  I_st : Inport
  Constant : Constant  Value=n_cell
  Constant1 : Constant  Value=M_v
  Constant2 : Constant  Value=F
  Constant3 : Constant  Value=M_O2
  MATLAB Function : MATLAB Function  TreatAsAtomicUnit=on
  MATLAB Function1 : MATLAB Function  TreatAsAtomicUnit=on
  W_O2_reac : Outport
  W_v_gen : Outport  Port=2
  wires:
  I_st/1 -> MATLAB Function1/1(I_st), MATLAB Function/1(I_st)
  MATLAB Function/1(W_O2_reac) -> W_O2_reac/1
  MATLAB Function1/1(W_v_gen) -> W_v_gen/1
  Constant/1 -> MATLAB Function/2(n_cell), MATLAB Function1/2(n_cell)
  Constant1/1 -> MATLAB Function1/3(M_v)
  Constant2/1 -> MATLAB Function/4(F), MATLAB Function1/4(F)
  Constant3/1 -> MATLAB Function/3(M_O2)

== system FM_V6_Zikun/Subsystem/FuelCellStack1/CathodMassFlow/InletFlowPropertiesCalc ==
  Phi_ca_in : Inport
  P_sat(T_ca_in) : Inport  Port=2
  P_ca_in : Inport  Port=3
  y_O2_ca_in : Inport  Port=4
  W_ca_in : Inport  Port=5
  3.40 : MATLAB Function  TreatAsAtomicUnit=on
  3.41 : MATLAB Function  TreatAsAtomicUnit=on
  3.42 : MATLAB Function  TreatAsAtomicUnit=on
  3.46 : MATLAB Function  TreatAsAtomicUnit=on
  Add : Sum  Inputs=+-
  Add1 : Sum  Inputs=+-
  Constant : Constant  Value=M_O2
  Constant1 : Constant  Value=M_N2
  Constant2 : Constant  Value=M_v
  Minus : Sum  Inputs=+-
  Product : Product
  Product1 : Product
  W_O2_ca_in : Outport
  W_N2_ca_in : Outport  Port=2
  W_v_ca_in : Outport  Port=3
  W_a_ca_in : Outport  Port=4
  tag scope: M_a_ca_in=global, w_ca_in=global
  wires:
  P_sat(T_ca_in)/1 -> Product/2
  Phi_ca_in/1 -> Product/1
  Product/1 -> 3.40/2(P_v_ca_in), Minus/2
  P_ca_in/1 -> Minus/1
  Minus/1 -> 3.40/3(P_a_ca_in)
  y_O2_ca_in/1 -> 3.46/1(y_O2_ca_in), 3.41/1(y_O2_ca_in)
  3.41/1(M_a_ca_in) -> 3.40/1(M_a_ca_in), [M_a_ca_in]
  3.40/1(w_ca_in) -> [w_ca_in], 3.42/2(w_ca_in)
  W_ca_in/1 -> Add/1, 3.42/1(W_ca_in)
  3.42/1(W_a_ca_in) -> Add/2, W_a_ca_in/1, Add1/1, Product1/1
  3.46/1(x_O2_ca_in) -> Product1/2
  Product1/1 -> Add1/2, W_O2_ca_in/1
  Add1/1 -> W_N2_ca_in/1
  Add/1 -> W_v_ca_in/1
  Constant/1 -> 3.46/2(M_O2), 3.41/2(M_O2)
  Constant1/1 -> 3.41/3(M_N2), 3.46/3(M_N2)
  Constant2/1 -> 3.40/4(M_v)

== system FM_V6_Zikun/Subsystem/FuelCellStack1/CathodMassFlow/OutletFlowPropertiesCalc ==
  W_ca_out : Inport
  P_sat(T_st) : Inport  Port=2
  P_O2_ca : Inport  Port=3
  Phi_ca : Inport  Port=4
  P_a_ca : Inport  Port=5
  3.48a : MATLAB Function  TreatAsAtomicUnit=on
  3.48b : MATLAB Function  TreatAsAtomicUnit=on
  3.48c : MATLAB Function  TreatAsAtomicUnit=on
  3.48e : MATLAB Function  TreatAsAtomicUnit=on
  Add : Sum  Inputs=+-
  Add1 : Sum  Inputs=+-
  Constant : Constant  Value=M_O2
  Constant1 : Constant  Value=M_N2
  Constant2 : Constant  Value=M_v
  P_v_ca : Product
  Product1 : Product
  y_O2_ca : Product  Inputs=*/
  W_O2_ca_out : Outport
  W_N2_ca_out : Outport  Port=2
  W_v_ca_out : Outport  Port=3
  W_a_ca_out : Outport  Port=4
  wires:
  P_a_ca/1 -> 3.48b/3(P_a_ca), y_O2_ca/2
  y_O2_ca/1 -> 3.48a/1(y_O2_ca), 3.48e/1(y_O2_ca)
  3.48a/1(M_a_ca) -> 3.48b/1(M_a_ca)
  3.48b/1(w_ca_out) -> 3.48c/2(w_ca_out)
  3.48c/1(W_a_ca_out) -> Add/2, Add1/1, W_a_ca_out/1, Product1/1
  3.48e/1(x_O2_ca) -> Product1/2
  Product1/1 -> Add1/2, W_O2_ca_out/1
  Add1/1 -> W_N2_ca_out/1
  Add/1 -> W_v_ca_out/1
  P_O2_ca/1 -> y_O2_ca/1
  Phi_ca/1 -> P_v_ca/1
  P_sat(T_st)/1 -> P_v_ca/2
  P_v_ca/1 -> 3.48b/2(P_v_ca)
  W_ca_out/1 -> 3.48c/1(W_ca_out), Add/1
  Constant2/1 -> 3.48b/4(M_v)
  Constant1/1 -> 3.48a/3(M_N2), 3.48e/3(M_N2)
  Constant/1 -> 3.48a/2(M_O2), 3.48e/2(M_O2)

== system FM_V6_Zikun/Subsystem/FuelCellStack1/CathodMassFlow/ThermodynamicCalc ==
  m_O2_ca : Inport
  m_N2_ca : Inport  Port=2
  m_v_ca : Inport  Port=3
  P_sat(T_st) : Inport  Port=4
  T_st : Inport  Port=5
  3.31 : MATLAB Function  TreatAsAtomicUnit=on
  3.32 : MATLAB Function  TreatAsAtomicUnit=on
  3.33 : MATLAB Function  TreatAsAtomicUnit=on
  3.34 : Sum
  3.35 : Sum  Inputs=+++
  3.37 : Product  Inputs=*/
  Constant : Constant  Value=V_ca
  Constant1 : Constant  Value=R_O2
  Constant2 : Constant  Value=R_N2
  Constant3 : Constant  Value=R_v
  P_ca : Outport
  P_a_ca : Outport  Port=2
  Phi_ca : Outport  Port=3
  P_O2_Ca : Outport  Port=4
  wires:
  Constant2/1 -> 3.32/2(R_N2)
  3.31/1(P_O2_Ca) -> P_O2_Ca/1, 3.34/1, 3.35/1
  Constant1/1 -> 3.31/2(R_O2)
  Constant3/1 -> 3.33/2(R_v)
  Constant/1 -> 3.31/4(V_ca), 3.32/4(V_ca), 3.33/4(V_ca)
  3.37/1 -> Phi_ca/1
  m_v_ca/1 -> 3.33/1(m_v_ca)
  T_st/1 -> 3.33/3(T_st), 3.31/3(T_st), 3.32/3(T_st)
  P_sat(T_st)/1 -> 3.37/2
  3.32/1(P_N2_Ca) -> 3.34/2, 3.35/2
  3.33/1(P_v_Ca) -> 3.37/1, 3.35/3
  m_O2_ca/1 -> 3.31/1(m_O2_ca)
  m_N2_ca/1 -> 3.32/1(m_N2_ca)
  3.35/1 -> P_ca/1
  3.34/1 -> P_a_ca/1

== system FM_V6_Zikun/Subsystem/FuelCellStack1/StackVoltage/ActivationLoss ==
  T_st : Inport
  P_ca : Inport  Port=2
  P_sat : Inport  Port=3
  P_O2 : Inport  Port=4
  I_den : Inport  Port=5
  ActivitionLoss : MATLAB Function  TreatAsAtomicUnit=on
  Constant : Constant  Value=c1
  MATLAB Function : MATLAB Function  TreatAsAtomicUnit=on
  MATLAB Function1 : MATLAB Function  TreatAsAtomicUnit=on
  MATLAB Function2 : MATLAB Function  TreatAsAtomicUnit=on
  V_act : Outport
  wires:
  ActivitionLoss/1(V_act) -> V_act/1
  MATLAB Function/1(V0) -> MATLAB Function2/1(V0), ActivitionLoss/1(V0)
  MATLAB Function1/1(Va) -> ActivitionLoss/2(Va), MATLAB Function2/2(Va)
  Constant/1 -> MATLAB Function2/3(c1), ActivitionLoss/3(c1)
  T_st/1 -> MATLAB Function1/1(T_st), MATLAB Function/1(T_st)
  P_ca/1 -> MATLAB Function/2(P_ca)
  P_sat/1 -> MATLAB Function1/3(P_sat), MATLAB Function/3(P_sat)
  P_O2/1 -> MATLAB Function1/2(P_O2)
  I_den/1 -> MATLAB Function2/4(I_den), ActivitionLoss/4(I_den)
  MATLAB Function2/1(R_act) -> [R_act]

== system FM_V6_Zikun/Subsystem/FuelCellStack1/StackVoltage/ConcentrationLoss ==
  I_den : Inport
  T_st : Inport  Port=2
  P_O2 : Inport  Port=3
  P_sat : Inport  Port=4
  Constant1 : Constant  Value=i_max
  Constant2 : Constant  Value=c3
  MATLAB Function : MATLAB Function  TreatAsAtomicUnit=on
  MATLAB Function1 : MATLAB Function  TreatAsAtomicUnit=on
  MATLAB Function2 : MATLAB Function  TreatAsAtomicUnit=on
  V_conc : Outport
  wires:
  I_den/1 -> MATLAB Function/1(I_den), MATLAB Function2/2(I_den)
  Constant2/1 -> MATLAB Function2/4(c3), MATLAB Function/4(c3)
  Constant1/1 -> MATLAB Function2/3(i_max), MATLAB Function/3(i_max)
  MATLAB Function1/1(c2) -> MATLAB Function2/1(c2), MATLAB Function/2(c2)
  MATLAB Function/1(V_conc) -> V_conc/1
  T_st/1 -> MATLAB Function1/1(T_st)
  P_O2/1 -> MATLAB Function1/2(P_O2)
  P_sat/1 -> MATLAB Function1/3(P_sat)
  MATLAB Function2/1(R_conc) -> [R_conc]

== system FM_V6_Zikun/Subsystem/FuelCellStack1/StackVoltage/OhmicLoss ==
  I_den : Inport
  T_st : Inport  Port=2
  lambda_m : Inport  Port=3
  Constant : Constant  Value=t_m
  Constant1 : Constant  Value=b11
  Constant2 : Constant  Value=b12
  Constant3 : Constant  Value=b2
  MATLAB Function : MATLAB Function  TreatAsAtomicUnit=on
  V_ohm : Outport
  wires:
  I_den/1 -> MATLAB Function/1(I_den)
  T_st/1 -> MATLAB Function/2(T_st)
  lambda_m/1 -> MATLAB Function/3(lambda_m)
  MATLAB Function/1(V_ohm) -> V_ohm/1
  Constant/1 -> MATLAB Function/4(t_m)
  Constant1/1 -> MATLAB Function/5(b11)
  Constant2/1 -> MATLAB Function/6(b12)
  Constant3/1 -> MATLAB Function/7(b2)

== system FM_V6_Zikun/Subsystem/FuelCellStack1/StackVoltage/VoltageBehaviour ==

== matlab function FM_V6_Zikun/Subsystem/Humidifier/2.39 ==
  data: W_cl input; W_v_cl output; W_a_cl input
function W_v_cl = fcn(W_cl, W_a_cl)

W_v_cl = W_cl - W_a_cl;

== matlab function FM_V6_Zikun/Subsystem/Humidifier/4.1 ==
  data: Phi_des input; W_v_inj output; P_sat_T_cl input; P_a_cl input; W_a_cl input; W_v_cl input; M_v input; M_a input
function W_v_inj = fcn(Phi_des, P_sat_T_cl, P_a_cl, W_a_cl, W_v_cl, M_v, M_a)

W_v_inj = ((M_v/M_a)*((Phi_des*P_sat_T_cl)/P_a_cl)*W_a_cl)-W_v_cl;

== matlab function FM_V6_Zikun/Subsystem/Humidifier/4.2 ==
  data: W_cl input; W_ca_in output; W_v_inj input
function W_ca_in = fcn(W_cl, W_v_inj)

W_ca_in = W_cl + W_v_inj;

== matlab function FM_V6_Zikun/Subsystem/Humidifier/4.3 ==
  data: P_a_cl input; P_ca_in output; Phi_des input; p_sat_T_cl input
function P_ca_in = fcn(P_a_cl, Phi_des, p_sat_T_cl)

P_ca_in = P_a_cl + Phi_des*p_sat_T_cl;

== matlab function FM_V6_Zikun/Subsystem/Tank/MATLAB Function ==
  data: m_w_tank input; cmd_refill output
function cmd_refill = fcn(m_w_tank)

cmd_refill = 0;
if m_w_tank == 0
    cmd_refill = 1;
end

== matlab function FM_V6_Zikun/Subsystem/Blower/MATLAB Function ==
  data: rho_H2 input; rho_N2 input; W_H2_tank input; W_an_in output; lambda_H2 input; ny_blower input; H2_ratio input; W_an_out output; P_an_in input; P_an input; P_blower output
function [W_an_in, W_an_out, P_blower] = fcn(rho_H2, rho_N2, W_H2_tank, lambda_H2, ny_blower, H2_ratio, P_an_in, P_an)

W_an_in = W_H2_tank*lambda_H2; % Flow to the anode [kg/s]

W_an_out = W_an_in - W_H2_tank; % Flow from the anode [kg/s]

delta_P_an = P_an_in-P_an; % Pressure difference over anode [Pa]

rho_an = H2_ratio*rho_H2 + (1-H2_ratio)*rho_N2; % Density of anode media [kg/m3]

P_blower = (delta_P_an*W_an_in/rho_an)/ny_blower; % Power consumption of [W]

== matlab function FM_V6_Zikun/Subsystem/Subsystem/MATLAB Function ==
  data: m_H2 input; P_H2_manifold output; R_H2 input; T_rm input; V_H2_manifold input
function P_H2_manifold = fcn(m_H2, R_H2,T_rm,V_H2_manifold)

P_H2_manifold = m_H2*R_H2*T_rm/V_H2_manifold;

== matlab function FM_V6_Zikun/Subsystem/Subsystem2/Subsystem/MATLAB Function3 ==
  data: W_cl output; T_st_ref input; T_st input; e_fan output
function [W_cl,e_fan] = fcn(T_st_ref,T_st)

e_fan = 0;
W_cl = 0.2*T_st-0.2*(T_st_ref-20);
if T_st <= T_st_ref-20
    e_fan = 0;
elseif (T_st_ref-20 < T_st) && T_st <= T_st_ref
    e_fan = 0;
elseif T_st > T_st_ref
    e_fan = T_st_ref - T_st;
end

== matlab function FM_V6_Zikun/Subsystem/Hydrogen Tank // Hydrogen Valve // Regulator1/MATLAB Function1 ==
  data: R_H2 input; V_tank input; P_tank output; T_tank input; P_tank_nom input; n_consumed input
function P_tank = fcn(R_H2, V_tank, T_tank, P_tank_nom, n_consumed)

n_tank_nom = P_tank_nom*V_tank/(R_H2*T_tank); % Nominal number of moles in tank, [n]

n_tank = n_tank_nom-n_consumed; % Moles in tank, [n]

P_tank = n_tank*R_H2*T_tank/V_tank; % Pressure in tank [Pa]

== matlab function FM_V6_Zikun/Subsystem/Subsystem2/Subsystem/MATLAB Function ==
  data: W_cl input; W_a input; T_cl_in input; nu_rad input; P_cl output; Cp_a input; Cp_cl input; T_a_in input
function P_cl = fcn(W_cl, W_a, T_cl_in, nu_rad, Cp_a, Cp_cl, T_a_in)

P_max_cl = Cp_cl*W_cl*(T_cl_in-T_a_in);
P_max_a = Cp_a*W_a*(T_cl_in-T_a_in);

P_max = (P_max_cl+P_max_a)/2;

P_cl = nu_rad*P_max;

== matlab function FM_V6_Zikun/Subsystem/Air Cooler/MATLAB Function ==
  data: P_cl input; phi_cl output; T_cl output; psat_Tcl output; P_a input; T_a input; phi_a input; T_cl input
function [phi_cl, T_cl, psat_Tcl] = fcn(P_cl, P_a, T_a,phi_a,T_cl) %p_cl=p_sm


psat_Ta = exp(20.386-5132/T_a)*133.3;
psat_Tcl = exp(20.386-5132/T_cl)*133.3;

phi_cl= (P_cl*phi_a*psat_Ta)/(P_a*psat_Tcl);

== matlab function FM_V6_Zikun/Subsystem/Subsystem2/Subsystem/MATLAB Function1 ==
  data: W_a input; P_fan_loss output; P_pump_loss output; W_cl input
function [P_fan_loss, P_pump_loss] = fcn(W_a, W_cl)

P_pump_loss = W_cl*80; % 80 W/(kg/s) from spec sheet
P_fan_loss= W_a*221; % 221 W/(kg/s) from spec sheet

== matlab function FM_V6_Zikun/Subsystem/Subsystem2/ThermoCalc/P_conv ==
  data: k_conv input; P_conv output; A_st input; T_a input; T_st input
function P_conv= fcn(k_conv,A_st,T_a,T_st)

P_conv = k_conv*A_st*(T_st-T_a);

== matlab function FM_V6_Zikun/Subsystem/AirExhaustManifold/MATLAB Function ==
  data: W_ca_out input; dP_rm output; W_rm_out input; R_a input; V_rm input; T_rm input
function dP_rm = fcn(W_ca_out,W_rm_out,R_a,V_rm,T_rm)

dP_rm = (W_ca_out-W_rm_out)*R_a*T_rm/V_rm;

== matlab function FM_V6_Zikun/Subsystem/Subsystem2/ThermoCalc/P_tot ==
  data: I_st input; P_tot output; F input; n_cell input
function P_tot = fcn(I_st,F,n_cell)

deltaH = -285.5;
P_tot = -(n_cell*I_st)/(2*F)*deltaH*1000;

== matlab function FM_V6_Zikun/Subsystem/AirExhaustManifold/MATLAB Function1 ==
  data: P_rm input; W_rm_out output; Cd_rm input; A_T_rm input; T_rm input; gamma input; R input; P_a input
function W_rm_out = fcn(P_rm,Cd_rm,A_T_rm,T_rm,gamma,R,P_a)

v1 = P_a/P_rm;
v2 = (2/(gamma+1))^(gamma/(gamma-1));

if  v1 >  v2
    W_rm_out = Cd_rm*A_T_rm*P_rm/sqrt(R*T_rm)*(P_a/P_rm)^(1/gamma)*(2*gamma/(gamma-1)*(1-(P_a/P_rm)^((gamma-1)/gamma)))^0.5;
else
    W_rm_out = Cd_rm*A_T_rm*P_rm/sqrt(R*T_rm)*gamma^0.5*(2/(gamma+1))^((gamma+1)/(2*(gamma-1)));
end

== matlab function FM_V6_Zikun/Subsystem/FuelCellStack1/StackVoltage/MATLAB Function ==
  data: E_T_P input; V_cell output; V_act input; V_ohm input; V_conc input
function V_cell = fcn(E_T_P,V_act,V_ohm,V_conc)

V_loss = V_act+V_ohm+V_conc;
if V_loss > E_T_P
    V_cell = 0;
else
    V_cell = E_T_P-V_loss;
end

== matlab function FM_V6_Zikun/Subsystem/Compressor/Subsystem/MATLAB Function ==
  data: M_v input; phi_a input; P_cp_in input; T_cp_in input; I_st input; W_cp output; n_cell input; F input; y_O2_ca_in input; O2_ER input; M_a_ca_in input; W_O2_ref output; M_O2 input
function [W_cp,W_O2_ref ]= fcn(M_v, phi_a, P_cp_in,T_cp_in,I_st,n_cell,F,y_O2_ca_in,O2_ER,M_a_ca_in,M_O2)


P_sat_a = exp(20.386-5132/T_cp_in)*133.3;
P_a_comp_in = P_cp_in - phi_a * P_sat_a;
P_v_cpmp_in = phi_a *P_sat_a;
w_cp_in = (M_v * P_v_cpmp_in)/(M_a_ca_in*P_a_comp_in);
W_cp = O2_ER*(1+w_cp_in)*(n_cell*I_st/(4*F))*(M_a_ca_in/y_O2_ca_in);
W_O2_ref=O2_ER*(n_cell*I_st/(4*F))*M_O2;

== matlab function FM_V6_Zikun/Subsystem/Compressor/Power calc 2/MATLAB Function ==
  data: gamma input; Power_cp output; P_cp_in input; W_ca_in input; rho_a input; copratio input
function Power_cp = fcn(gamma,P_cp_in,W_ca_in,rho_a,copratio)

Power_cp = (gamma/(gamma-1)) * P_cp_in * (W_ca_in/rho_a) * (1 -( copratio  ^ ((gamma-1)/gamma)))   ;

== matlab function FM_V6_Zikun/Subsystem/FuelCellStack1/Anode Flow Model/Diffusion/H2 Crossflow ==
  data: n_cell input; W_H2_an_cf output; A_fc input; t_m input; P_an input; W_H2_an_in input; T_st input; W_H2_an_in2 output
function [W_H2_an_cf, W_H2_an_in2]= fcn(n_cell, A_fc, t_m, P_an, W_H2_an_in, T_st)

D_H2 = 0.0041*exp(-2602/T_st); % Diffusivity, cm^2/s (4.17)
S_H2 = 2.2E-10; % Solubility, mol/(cm^3*Pa)

P_H2 = D_H2*S_H2; % Permeability, mol*cm/(s*cm^2*Pa) (4.16)

W_H2_an_cf = P_H2*n_cell*A_fc*P_an/t_m*2.016E-3; % Cross flow

W_H2_an_in2 = W_H2_an_in - W_H2_an_cf; % Remaining hydrogen flow

== matlab function FM_V6_Zikun/Subsystem/FuelCellStack1/Anode Flow Model/InletFlow/anode humidity ratio (3.62) ==
  data: P_v_an_in input; w_an_in output; P_an_in input; M_v input; M_H2 input
function w_an_in = fcn(P_v_an_in,P_an_in,M_v,M_H2)

w_an_in= M_v*P_v_an_in/(M_H2*P_an_in);

== matlab function FM_V6_Zikun/Subsystem/FuelCellStack1/Anode Flow Model/InletFlow/mass flow rates of hydrogen (3.63) ==
  data: w_an_in input; W_H2_an_in output; W_an_in input
function W_H2_an_in = fcn(w_an_in,W_an_in)

W_H2_an_in = W_an_in/(1+w_an_in);

== matlab function FM_V6_Zikun/Subsystem/Supply Manifold/Manifold Filling/MATLAB Function2 ==
  settings: updateMethod=DISCRETE
  data: m_sm input; T_sm output; p_sm input; V_sm input; R_a input
function T_sm = fcn(m_sm, p_sm,V_sm,R_a)

    %V_sm = 0.02; %m3
    %Ra = 286.9; %J/KgK

    persistent firstit

    if isempty(firstit)
        firstit = true;
    end

    if firstit
        T_sm = 400;
        firstit = false; % Set firstit to false after the first iteration
    else
        T_sm = (p_sm*V_sm)/(m_sm*R_a);
    end
end

== matlab function FM_V6_Zikun/Subsystem/FuelCellStack1/Anode Flow Model/InletFlow/rate of hydrogen consumed in the reaction (3.65) ==
  data: I_st input; W_H2_reacted output; n_cell input; M_H2 input; F input
function W_H2_reacted = fcn(I_st,n_cell,M_H2,F)

W_H2_reacted = M_H2*n_cell*I_st/(2*F);

== matlab function FM_V6_Zikun/Subsystem/FuelCellStack1/Anode Flow Model/MassBalance/3.51 ==
  data: W_H2_an_in input; dm_H2_an output; W_H2_an_out input; W_H2_reac input
function dm_H2_an = fcn(W_H2_an_in,W_H2_an_out,W_H2_reac)

dm_H2_an = W_H2_an_in-W_H2_an_out-W_H2_reac;

== matlab function FM_V6_Zikun/Subsystem/FuelCellStack1/Anode Flow Model/MassBalance/3.52 ==
  data: W_v_an_in input; dm_w_an output; W_v_an_out input; W_v_mem input; W_l_an_out input
function dm_w_an = fcn(W_v_an_in,W_v_an_out,W_v_mem,W_l_an_out)

dm_w_an = W_v_an_in-W_v_an_out-W_v_mem-W_l_an_out;

== matlab function FM_V6_Zikun/Subsystem/FuelCellStack1/Anode Flow Model/MassBalance/3.53 & 3.54 ==
  data: m_v_max_an input; m_w_an input; m_v_an output; m_l_an output
function [m_v_an, m_l_an]= fcn(m_v_max_an,m_w_an)

if m_w_an <= m_v_max_an
    m_v_an=m_w_an;
    m_l_an=0;
else
    m_v_an=m_v_max_an;
    m_l_an=m_w_an-m_v_max_an;
end

== matlab function FM_V6_Zikun/Subsystem/FuelCellStack1/Anode Flow Model/MassBalance/maximum vapor mass (3.55) ==
  data: p_sat_tst input; m_v_max_an output; T_st input; V_an input; R_v input
function m_v_max_an = fcn(p_sat_tst,T_st,V_an,R_v)

m_v_max_an = p_sat_tst*V_an/(R_v*T_st);
